simulink model "doc_design_iteration_viterbi_rayleigh_OFDM"  (R2014a)
settings: Solver=FixedStepDiscrete  SolverMode=SingleTasking  StartTime=0.0  StopTime=inf  RelTol=1e-3
PostLoadFcn:
  | if ~exist('EbNo'),EbNo=6;end
  | if ~exist('maxNumBits'),maxNumBits=1e7;end;
  | if ~exist('maxNumErrs'),maxNumErrs=1e3;end;
  | if ~exist('Seed'),Seed=211;end;
  | 
  | Param.BitsPerFrame=186;
  | Param.Len1=186+6;
  | pre1=0.5*((-1).^(0:1:99)+1);
  | pre2=0.5*((-1).^(1:100)+1);
  | Param.Preamble=complex([pre1 0.0 pre2].');
  | 
  | clear pre1 pre2
values from neighbouring files (symbols this model uses):
  EbNo = getTestParameter(obj,'EbNo')    [GrayCodedMod_EbNo_M.m]    (also in GrayCodedModulation2.m; commdoc_code.m = 10; commdoc_gray.m = 10; commdoc_mcurves.m = EbNoVec(idxEbNo))
undefined symbols (not defined in the file or in its folder): magnitude
libraries: dspindex x3, commchan3 x2, dspmtrx3 x2, commdigbbndpm3 x2, commofdm x2, commcnvcod2 x2, dspstat3 x1, dspmathops x1, dspsigops x1, commsink2 x1, commrandsrc2 x1
settings Model: Creator=The MathWorks Inc.
settings OptimizationCC: ExpressionDepthLimit=2147483647
settings DebuggingCC: UnderspecifiedInitializationDetection=Classic  SolverPrmCheckMsg=none  StateNameClashWarn=warning

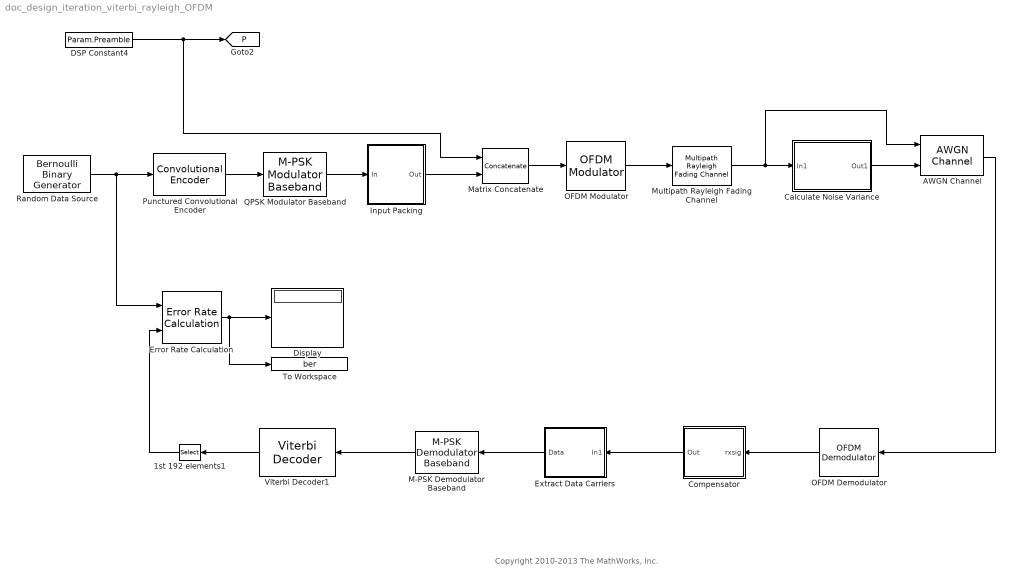
== system doc_design_iteration_viterbi_rayleigh_OFDM ==
  note: Copyright 2010-2013 The MathWorks, Inc.
  1st 192 elements1 : Selector  NumberOfDimensions=2  InputPortWidth=3  IndexOptions=Index vector (dialog),Index vector (dialog)  Indices=1:186,1  OutputSizes=1,1
  AWGN Channel : commchan3/AWGN Channel  InputProcessing=Columns as channels (frame based)  seed=67  noiseMode=Variance from port  EbNodB=10  EsNodB=15  SNRdB=10  bitsPerSym=1  Ps=1  Tsym=1e-6  variance=1
  Calculate Noise Variance : Subsystem
      mask Display: disp('Calculate\nNoise Variance')
  Compensator : Subsystem
      mask Display: disp('Gain & Phase\nCompensator');
  DSP Constant4 : Constant  Value=Param.Preamble  VectorParams1D=off
      settings: SamplingMode=Frame based
  Display : Display
  Error Rate Calculation : commsink2/Error Rate Calculation  N=0  st_delay=0  cp_mode=Entire frame  subframe=[]  PMode=Port  WsName=ErrorVec1  RsMode2=off  stop=on  numErr=maxNumErrs  maxBits=maxNumBits
  Extract Data Carriers : Subsystem
      mask Display: disp('Extract\nData Carriers');
  Input Packing : Subsystem
      mask Display: disp('IFFT Input\nPacking');
  M-PSK Demodulator Baseband : commdigbbndpm3/M-PSK Demodulator Baseband  M=4  Ph=pi/4  Dec=Gray  Mapping=[0 2 3 1]  OutType=Bit  DecType=Hard decision  VarSource=Dialog  Variance=1  outDtype1=boolean  outDtype2=Inherit via internal rule  derotateFactorWordLen=16
  Matrix Concatenate : Concatenate  Mode=Multidimensional array  ConcatenateDimension=2
  Multipath Rayleigh Fading Channel : commchan3/Multipath Rayleigh Fading Channel  maxDopplerShift=5  spectrumType=Jakes  sigmaGaussian=1/sqrt(2)  coeffRounded=[1 -1.72 0.785]  freqMinMaxRJakes=[0 1]  freqMinMaxAJakes=[0 1]  sigmaGaussian1=1/sqrt(2)  sigmaGaussian2=1/sqrt(2)  centerFreqGaussian1=0.0  centerFreqGaussian2=0.0  gainGaussian1=0.5  gainGaussian2=0.5  coeffBell=9  dopplerSpectrum=doppler.jakes  pathDelays=[0 0.4 0.9]*1e-6  avgPathGaindB=[0 -5 -10]  normalizePathGains=on  seed=211  enableProbe=0  openVisAtStart=off  outPathGains=off  outDelay=off
  OFDM Demodulator : commofdm/OFDM Demodulator  SimulateUsing=Code generation  FFTLength=256  NumGuardBandCarriers=[27;27]  RemoveDCCarrier=on  PilotOutputPort=off  PilotCarrierIndices=[12; 26; 40; 54]  CyclicPrefixLength=32  NumSymbols=2  NumReceiveAntennas=1
  OFDM Modulator : commofdm/OFDM Modulator  SimulateUsing=Code generation  FFTLength=256  NumGuardBandCarriers=[27;27]  InsertDCNull=on  PilotInputPort=off  PilotCarrierIndices=[12; 26; 40; 54]  CyclicPrefixLength=32  Windowing=off  WindowLength=1  NumSymbols=2  NumTransmitAntennas=1
  Punctured Convolutional Encoder : commcnvcod2/Convolutional Encoder  trellis=poly2trellis(7, [171 133])  opMode=Terminate trellis by appending bits  DelayedResetAction=off  hasIniStPort=off  hasFinStPort=off  usePuncVector=on  punctureVector=reshape([1 0;1 1],4,1)  reset=Unused parameter value
  QPSK Modulator Baseband : commdigbbndpm3/M-PSK Modulator Baseband  M=4  InType=Bit  Enc=Gray  Mapping=[0 2 3 1]  Ph=pi/4  outDtype=double  outWordLen=16  outUDDataType=sfix(16)  outFracLenMode=Best precision  outFracLen=15
  Random Data Source : commrandsrc2/Bernoulli Binary Generator  P=0.5  seed=61  Ts=25/3e6  frameBased=on  sampPerFrame=186  orient=off  outDataType=boolean
  To Workspace : ToWorkspace  VariableName=ber  SampleTime=-1
      settings: MaxDataPoints=1
  Viterbi Decoder1 : commcnvcod2/Viterbi Decoder  trellis=poly2trellis(7, [171 133])  isPunctured=off  punctureVector=reshape([1 0;1 1],4,1)  erasures=off  dectype=Hard decision  runSigValErrCheck=off  nsdecb=4  smWordLength=16  tbdepth=34  opmode=Terminated  reset=off  outDataType=boolean  delayedResetAction=off
  tag scope: P=global
  wires:
  Random Data Source/1 -> Error Rate Calculation/1, Punctured Convolutional Encoder/1
  Punctured Convolutional Encoder/1 -> QPSK Modulator Baseband/1
  QPSK Modulator Baseband/1 -> Input Packing/1(In)
  Multipath Rayleigh Fading Channel/1 -> AWGN Channel/1, Calculate Noise Variance/1(In1)
  DSP Constant4/1 -> Matrix Concatenate/1, [P]
  Compensator/1(Out) -> Extract Data Carriers/1(In1)
  Extract Data Carriers/1(Data) -> M-PSK Demodulator Baseband/1
  M-PSK Demodulator Baseband/1 -> Viterbi Decoder1/1
  Viterbi Decoder1/1 -> 1st 192 elements1/1
  Error Rate Calculation/1 -> Display/1, To Workspace/1
  1st 192 elements1/1 -> Error Rate Calculation/2
  OFDM Demodulator/1 -> Compensator/1(rxsig)
  Input Packing/1(Out) -> Matrix Concatenate/2
  Matrix Concatenate/1 -> OFDM Modulator/1
  OFDM Modulator/1 -> Multipath Rayleigh Fading Channel/1
  Calculate Noise Variance/1(Out1) -> AWGN Channel/2
  AWGN Channel/1 -> OFDM Demodulator/1

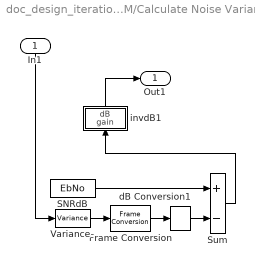
== system doc_design_iteration_viterbi_rayleigh_OFDM/Calculate Noise Variance ==
  In1 : Inport
  Frame Conversion : FrameConversion  OutFrame=Sample-based
  SNRdB : Constant  Value=EbNo
  Sum : Sum  Inputs=+-  SaturateOnIntegerOverflow=on
  Variance : dspstat3/Variance  run=off  reset_popup=None  InputProcessing=Columns as channels (frame based)  directionMode=Each column  dimension=1  treatSBRowAsCol=on  roiEnable=off  roiType=Rectangles  roiPortion=Entire ROI  roiOutput=Individual statistics for each ROI  roiFlag=off  roundingMode=Floor  overflowMode=off
  dB Conversion1 : dspmathops/dB Conversion  dBtype=dB  intype=Power  R=1  fuzz=on
  invdB1 : Subsystem
      mask Display: disp('1/invdB')
  Out1 : Outport
  wires:
  invdB1/1(dB) -> Out1/1
  Sum/1 -> invdB1/1(gain)
  SNRdB/1 -> Sum/1
  Variance/1 -> Frame Conversion/1
  Frame Conversion/1 -> dB Conversion1/1
  dB Conversion1/1 -> Sum/2
  In1/1 -> Variance/1

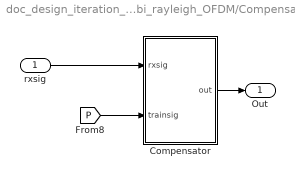
== system doc_design_iteration_viterbi_rayleigh_OFDM/Compensator ==
  rxsig : Inport
  Compensator : Subsystem
      mask init:
      | a = [1:100; 1:100];
      mask Display: disp('Gain & Phase\nCompensator')
  Out : Outport
  wires:
  Compensator/1(out) -> Out/1
  rxsig/1 -> Compensator/1(rxsig)
  [P] -> Compensator/2(trainsig)

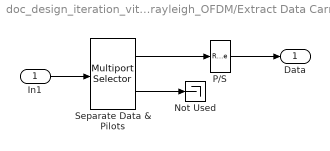
== system doc_design_iteration_viterbi_rayleigh_OFDM/Extract Data Carriers ==
  In1 : Inport
  Not Used : Terminator
  P/S : Reshape  OutputDimensionality=Column vector (2-D)  OutputDimensions=[72, 1]
  Separate Data & Pilots : dspindex/Multiport Selector  rowsOrCols=Rows  idxCellArray={[1:12 14:37 39:62 64:87 89:112 114:137 139:162 164:187 189:200],[13 38 63 88 113 138 163 188]}  idxErrMode=Clip Index
  Data : Outport
  wires:
  In1/1 -> Separate Data & Pilots/1
  Separate Data & Pilots/2 -> Not Used/1
  Separate Data & Pilots/1 -> P/S/1
  P/S/1 -> Data/1

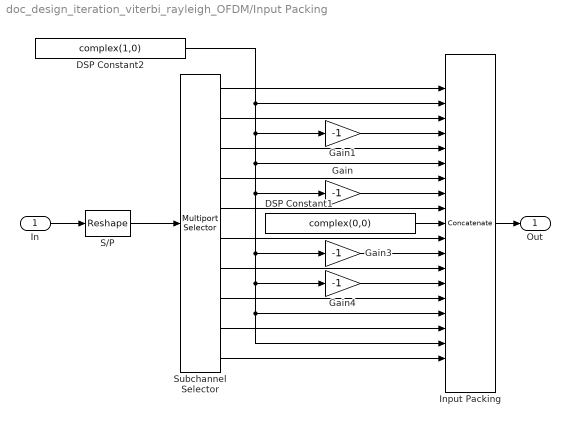
== system doc_design_iteration_viterbi_rayleigh_OFDM/Input Packing ==
  In : Inport
  DSP Constant1 : Constant  Value=complex(0,0)  VectorParams1D=off
      settings: SamplingMode=Frame based
  DSP Constant2 : Constant  Value=complex(1,0)  VectorParams1D=off  FramePeriod=Inf
      settings: SamplingMode=Frame based
  Gain{,1,3..4} (4 alike) : Gain  Gain=-1
  Input Packing : Concatenate  NumInputs=19  Mode=Multidimensional array
  S/P : Reshape  OutputDimensionality=Customize  OutputDimensions=[192,1]
  Subchannel Selector : dspindex/Multiport Selector  rowsOrCols=Rows  idxCellArray={[1:12],[13:36],[37:60],[61:84],[85:96],[97:108],[109:132],[133:156],[157:180],[181:192]}  idxErrMode=Generate Error
  Out : Outport
  wires:
  Input Packing/1 -> Out/1
  Gain4/1 -> Input Packing/14
  Gain3/1 -> Input Packing/12
  S/P/1 -> Subchannel Selector/1
  Gain1/1 -> Input Packing/4
  Gain/1 -> Input Packing/8
  DSP Constant1/1 -> Input Packing/10
  Subchannel Selector/1 -> Input Packing/1
  Subchannel Selector/2 -> Input Packing/3
  Subchannel Selector/3 -> Input Packing/5
  Subchannel Selector/4 -> Input Packing/7
  Subchannel Selector/5 -> Input Packing/9
  Subchannel Selector/6 -> Input Packing/11
  Subchannel Selector/7 -> Input Packing/13
  Subchannel Selector/8 -> Input Packing/15
  Subchannel Selector/9 -> Input Packing/17
  Subchannel Selector/10 -> Input Packing/19
  DSP Constant2/1 -> Input Packing/2, Input Packing/6, Gain3/1, Gain4/1, Input Packing/18, Input Packing/16, Gain/1, Gain1/1
  In/1 -> S/P/1

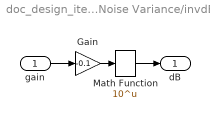
== system doc_design_iteration_viterbi_rayleigh_OFDM/Calculate Noise Variance/invdB1 ==
  gain : Inport
  Gain : Gain  Gain=-0.1  SaturateOnIntegerOverflow=on  OutDataTypeStr=Inherit: Same as input  ParamDataTypeStr=Inherit: Same as input
  Math Function : Math  Operator=10^u  SaturateOnIntegerOverflow=on
  dB : Outport
  wires:
  Gain/1 -> Math Function/1
  gain/1 -> Gain/1
  Math Function/1 -> dB/1

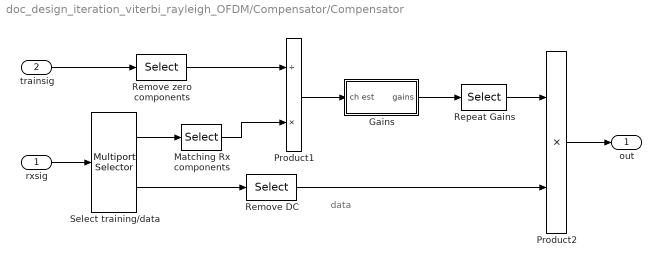
== system doc_design_iteration_viterbi_rayleigh_OFDM/Compensator/Compensator ==
  note: data
  rxsig : Inport
  trainsig : Inport  Port=2
  Gains : Subsystem
  Matching Rx components : Selector  NumberOfDimensions=2  InputPortWidth=53  IndexOptions=Index vector (dialog),Select all  Indices=[1:2:99 103:2:201],-1
  Product1 : Product  Inputs=/*  SaturateOnIntegerOverflow=on  OutDataTypeStr=Inherit: Same as first input
  Product2 : Product  Inputs=**  SaturateOnIntegerOverflow=on  OutDataTypeStr=Inherit: Same as first input
  "Remove DC " : Selector  NumberOfDimensions=2  InputPortWidth=53  IndexOptions=Index vector (dialog),Select all  Indices=[1:100 102:201],-1
  Remove zero components : Selector  NumberOfDimensions=2  InputPortWidth=53  IndexOptions=Index vector (dialog),Select all  Indices=[1:2:99 103:2:201],-1
  Repeat Gains : Selector  NumberOfDimensions=2  InputPortWidth=53  IndexOptions=Index vector (dialog),Select all  Indices=a(:),-1
  Select training/data : dspindex/Multiport Selector  rowsOrCols=Columns  idxCellArray={1,2}  idxErrMode=Clip Index
  out : Outport
  wires:
  "Remove DC "/1 -> Product2/2
  Repeat Gains/1 -> Product2/1
  Remove zero components/1 -> Product1/1
  rxsig/1 -> Select training/data/1
  Select training/data/2 -> "Remove DC "/1
  Gains/1(gains) -> Repeat Gains/1
  Product1/1 -> Gains/1(ch est)
  Select training/data/1 -> Matching Rx components/1
  trainsig/1 -> Remove zero components/1
  Product2/1 -> out/1
  Matching Rx components/1 -> Product1/2

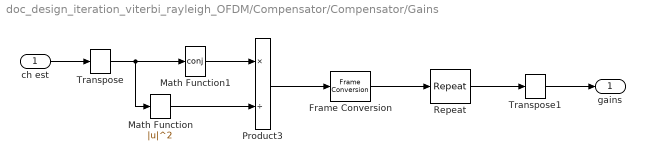
== system doc_design_iteration_viterbi_rayleigh_OFDM/Compensator/Compensator/Gains ==
  ch est : Inport
  Frame Conversion : FrameConversion
  Math Function : Math  Operator=magnitude^2  SaturateOnIntegerOverflow=on
  Math Function1 : Math  Operator=conj  SaturateOnIntegerOverflow=on
  Product3 : Product  Inputs=*/  SaturateOnIntegerOverflow=on  OutDataTypeStr=Inherit: Same as first input
  Repeat : dspsigops/Repeat  N=1  InputProcessing=Columns as channels (frame based)  RateOptions=Enforce single-rate processing  ic=0  mode=Unused parameter value
  Transpose : dspmtrx3/Transpose  Hermitian=off  overflowFlag=on
  Transpose1 : dspmtrx3/Transpose  Hermitian=off  overflowFlag=on
  gains : Outport
  wires:
  ch est/1 -> Transpose/1
  Math Function/1 -> Product3/2
  Math Function1/1 -> Product3/1
  Product3/1 -> Frame Conversion/1
  Transpose/1 -> Math Function1/1, Math Function/1
  Frame Conversion/1 -> Repeat/1
  Repeat/1 -> Transpose1/1
  Transpose1/1 -> gains/1
